simulink model "untitled"  (R2023b)
settings: Solver=VariableStepAuto  StartTime=0.0  StopTime=200.0  RelTol=1e-3
PreLoadFcn:
  | preload = "pre load";
  | disp(preload);
PostLoadFcn:
  | disp("hogehoge")
  | postload = "post load"
  | exist("post_load_function.m","file")
  | run("post_load_function.m");
InitFcn:
  | init = "init";
  | disp(init);
StartFcn:
  | start = "start";
  | disp(start);
values from neighbouring files (symbols this model uses):
  dt = 0.025    [9_26_1.mat]    (also in CONTROLLER_SYSTEM.m = obj.dt; Copy_of_drone_model.m = "double")
undefined symbols (not defined in the file or in its folder): drone_model
settings Model: Creator=kasek  LastModifiedBy=kasek

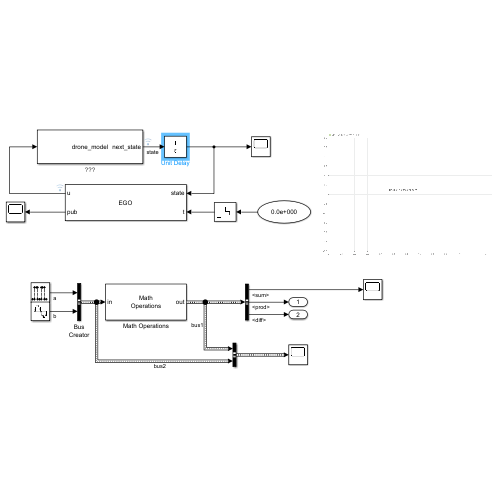
[thumbnail: Simulink's stored preview of the top-level diagram]
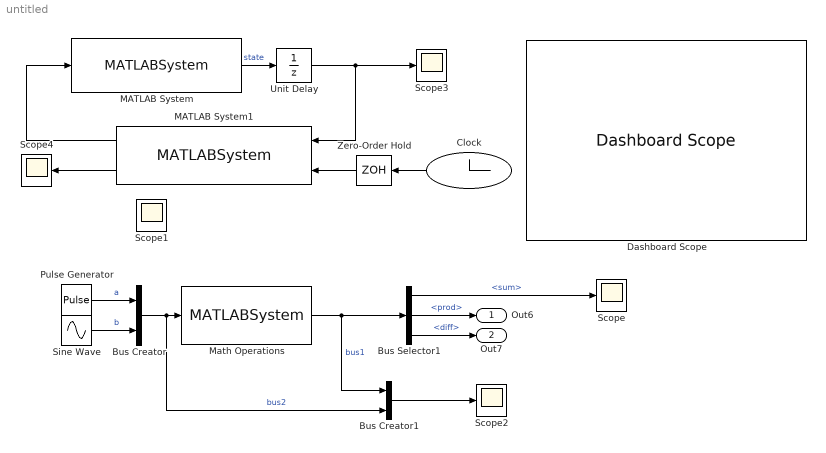
== system untitled ==
  Bus Creator : BusCreator  Inputs=2  OutDataTypeStr=Bus: mybus  NonVirtualBus=on
  Bus Creator1 : BusCreator  Inputs=2  OutDataTypeStr=Bus: my_Bus  NonVirtualBus=on
  Bus Selector1 : BusSelector  OutputSignals=sum,prod,diff
  Clock : Clock
  Dashboard Scope : DashboardScope
  MATLAB System : MATLABSystem  System=drone_model  SimulateUsing=Interpreted execution
      settings: AttributesFormatString=%<A>
      mask Type: drone_model
      mask Display:
      | disp('drone_model');
      | port_label('output',1,'next_state');
  MATLAB System1 : MATLABSystem  System=EGO  initial_control_signal=[ 0; 0; 0; 0 ]  SimulateUsing=Interpreted execution
      mask Type: EGO
      mask Display:
      | disp('EGO');
      | port_label('input',1,'state');
      | port_label('input',2,'t');
      | port_label('output',1,'u');
      | port_label('output',2,'pub');
  Math Operations : MATLABSystem  System=slexBusesMATLABSystemMathOpSysObj  SimulateUsing=Code generation
      mask Type: slexBusesMATLABSystemMathOpSysObj
      mask Display:
      | disp(['Math' char(10) 'Operations']);
      | port_label('input',1,'in');
      | port_label('output',1,'out');
  Pulse Generator : DiscretePulseGenerator
  Scope{,1..4} (5 alike) : Scope
  Sine Wave : Sin  SampleTime=1
  Unit Delay : UnitDelay  InitialCondition="drone_model.get(\"initial_state\")"  SampleTime=dt  HasFrameUpgradeWarning=on
  Zero-Order Hold : ZeroOrderHold  SampleTime=dt
  Out6 : Outport  VectorParamsAs1DForOutWhenUnconnected=off
  Out7 : Outport  Port=2  VectorParamsAs1DForOutWhenUnconnected=off
  wires:
  MATLAB System/1 -> Unit Delay/1  "state"
  Math Operations/1 -> Bus Creator1/1, Bus Selector1/1  "bus1"
  Bus Selector1/2 -> Out6/1  "<prod>"
  Bus Selector1/3 -> Out7/1  "<diff>"
  Bus Selector1/1 -> Scope/1  "<sum>"
  Bus Creator/1 -> Bus Creator1/2, Math Operations/1  "bus2"
  Sine Wave/1 -> Bus Creator/2  "b"
  Pulse Generator/1 -> Bus Creator/1  "a"
  Bus Creator1/1 -> Scope2/1
  Clock/1 -> Zero-Order Hold/1
  MATLAB System1/1 -> MATLAB System/1
  Zero-Order Hold/1 -> MATLAB System1/2
  MATLAB System1/2 -> Scope4/1
  Unit Delay/1 -> Scope3/1, MATLAB System1/1
